simulink model "deadbeatRegulator"  (R2013b)
settings: Solver=ode45  StartTime=0.0  StopTime=15  RelTol=1e-3
settings Model: Creator=Darko  LastModifiedBy=Darko

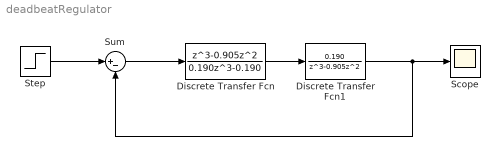
== system deadbeatRegulator ==
  Discrete Transfer Fcn : DiscreteTransferFcn  Numerator=[1 -0.905 0 0]  Denominator=[0.190 0 0 -0.190]  SampleTime=2
  Discrete Transfer Fcn1 : DiscreteTransferFcn  Numerator=[0.190]  Denominator=[1 -0.905 0 0]  SampleTime=2
  Scope : Scope
  Step : Step  Time=0  SampleTime=0.01
  Sum : Sum  Inputs=|+-
  wires:
  Step/1 -> Sum/1
  Sum/1 -> Discrete Transfer Fcn/1
  Discrete Transfer Fcn/1 -> Discrete Transfer Fcn1/1
  Discrete Transfer Fcn1/1 -> Sum/2, Scope/1
